simulink model "Lab_09_simulink"  (R2024b)
settings: Solver=VariableStepAuto  StartTime=0.0  StopTime=10.0  RelTol=1e-3
libraries: dspfdesign x1
settings Model: LastModifiedBy=LENOVO

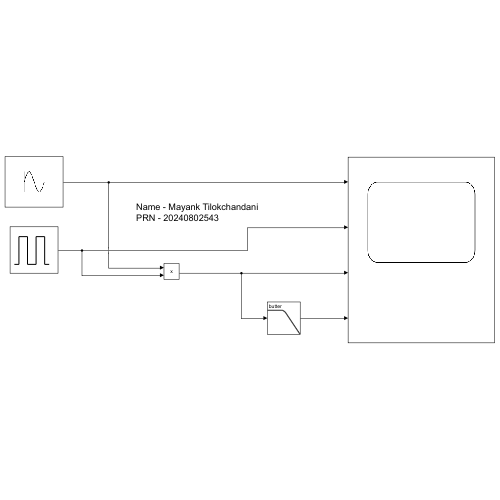
[thumbnail: Simulink's stored preview of the top-level diagram]
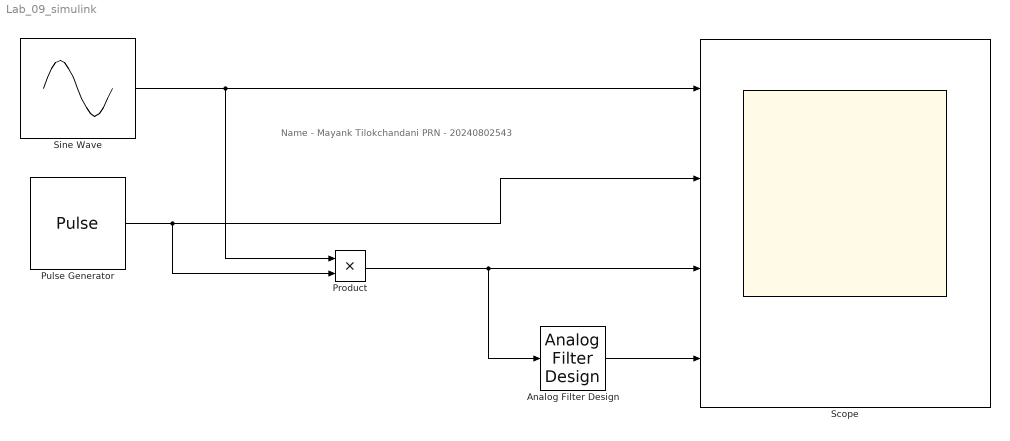
== system Lab_09_simulink ==
  note: Name - Mayank Tilokchandani
      | PRN - 20240802543
  Analog Filter Design : dspfdesign/Analog Filter Design  method=Butterworth  filttype=Lowpass  N=5  Wlo=4  Whi=80  Rp=2  Rs=40
  Product : Product
  Pulse Generator : DiscretePulseGenerator  PulseType=Time based  Amplitude=10  Period=0.6  PulseWidth=50
  Scope : Scope  NumInputPorts=4
  Sine Wave : Sin  SampleTime=0
  wires:
  Pulse Generator/1 -> Product/2, Scope/2
  Sine Wave/1 -> Product/1, Scope/1
  Product/1 -> Analog Filter Design/1, Scope/3
  Analog Filter Design/1 -> Scope/4
